simulink model "experience2"  (R2018b)
settings: Solver=VariableStepAuto  StartTime=0.0  StopTime=10.0  RelTol=1e-3
values from neighbouring files (symbols this model uses):
  b = 3.5077e-6    (= 3.5077e-06)    [experience2Extention.m]
  J = 3.2284e-5    (= 3.2284e-05)    [experience2Extention.m]
  K = 0.0274    [experience2Extention.m]
  L = 2.75e-6    (= 2.75e-06)    [experience2Extention.m]
  R = 4    [experience2Extention.m]
settings Model: Creator=Alireza  LastModifiedBy=Alireza

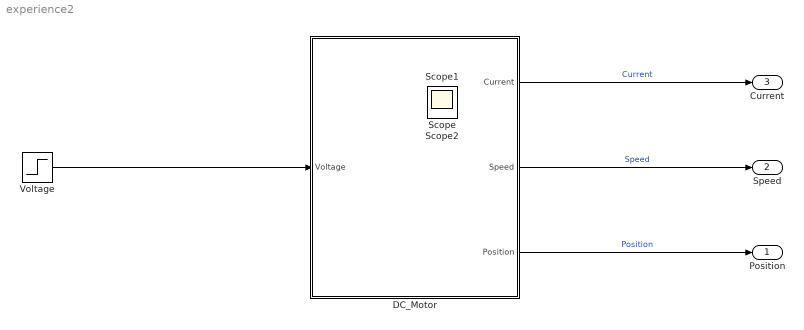
== system experience2 ==
  DC_Motor : Subsystem
  Voltage : Step  Time=0  SampleTime=0
  Position : Outport
  Speed : Outport  Port=2
  Current : Outport  Port=3
  Scope : Scope
  Scope1 : Scope
  Scope2 : Scope
  wires:
  Voltage/1 -> DC_Motor/1(Voltage)
  DC_Motor/1(Current) -> Current/1  "Current"
  DC_Motor/2(Speed) -> Speed/1  "Speed"
  DC_Motor/3(Position) -> Position/1  "Position"

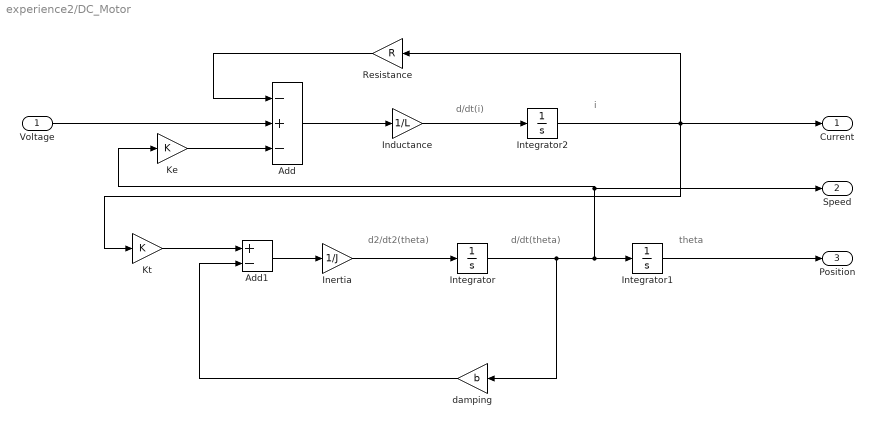
== system experience2/DC_Motor ==
  note: i
  note: d/dt(i)
  note: theta
  note: d/dt(theta)
  note: d2/dt2(theta)
  Voltage : Inport
  Add : Sum  Inputs=-+-
  Add1 : Sum  Inputs=+-
  Inductance : Gain  Gain=1/L
  Inertia : Gain  Gain=1/J
  Integrator : Integrator
  Integrator1 : Integrator
  Integrator2 : Integrator
  Ke : Gain  Gain=K
  Kt : Gain  Gain=K
  "Resistance " : Gain  Gain=R
  "damping " : Gain  Gain=b
  Current : Outport
  Speed : Outport  Port=2
  Position : Outport  Port=3
  wires:
  Inertia/1 -> Integrator/1
  Add/1 -> Inductance/1
  Voltage/1 -> Add/2
  Ke/1 -> Add/3
  Add1/1 -> Inertia/1
  Kt/1 -> Add1/1
  Inductance/1 -> Integrator2/1
  Integrator/1 -> "damping "/1, Speed/1, Ke/1, Integrator1/1
  "damping "/1 -> Add1/2
  Integrator2/1 -> Current/1, "Resistance "/1, Kt/1
  "Resistance "/1 -> Add/1
  Integrator1/1 -> Position/1
